simulink model "cblocks"  (Simulink 6.5)
settings: Solver=ode45  SolverMode=SingleTasking  StartTime=0.0  StopTime=999999  MaxStep=10  RelTol=1e-3  AbsTol=1e-3
undefined symbols (not defined in the file or in its folder): TSAMPLE, Upmax, Upmin
settings Model: Creator=Kostas Tsakalis  LastModifiedBy=Kostas Tsakalis
settings DataIOCC: LimitDataPoints=off  SaveOutput=off  SaveTime=off  SignalLoggingName=sigsOut
settings OptimizationCC: BooleanDataType=off
settings DebuggingCC: SolverPrmCheckMsg=none  MultiTaskDSMMsg=warning  MultiTaskCondExecSysMsg=none  StrictBusMsg=None
settings HardwareCC: TargetUnknown=on
settings RTWCC: IncludeERTFirstTime=on

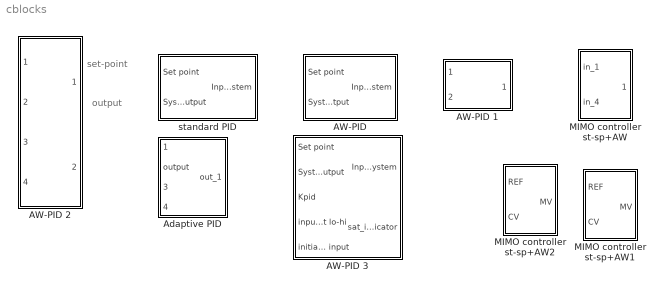
== system cblocks ==
  note: set-point
  note: output
  "AW-PID " : Subsystem  mask(Anti-windup PID ){@1=[.05, 3, 0.5], @2=1/60, @3=0.1, @4=1/60, @5=[0.7 -0.3]}
      mask prompts: @1 "Gain kp - Integral time ki - Derivative time kd"; @2 "Pseudo-derivative filter time constant"; @3 "Error lowpass filter Time constant"; @4 "Sampling Time"; @5 "Saturation Limits [umax umin]"
      mask help: Discrete PID with Anti-windup and with lowpass filter
      mask init:
      | kp=@1(1);ki=@1(2);kd=@1(3);SAM=@2;TF=@3;DT=@4;umax=@5(1);umin=@5(2);
      mask Display: disp('AW-PID+filter')
  AW-PID 1 : Subsystem  mask(Anti-windup PID ){SAM=10, DT=10}
      mask prompts: SAM "Gains: [proportional, Integral, Derivative]"; DT "Pseudo-derivative filter time constant"
      mask help: Discrete PID with Anti-windup
      mask init:
      | kp=@1(1);ki=@1(2);kd=@1(3);umax=@4(1);umin=@4(2);
      mask Display:
      | port_label('output',1,'u')
      | port_label('input',1,'r')
      | port_label('input',2,'y')
  AW-PID 2 : Subsystem  mask(Anti-windup PID ){kpid=[11, 30, 1.5], TCD=.01, TF=0, DT=.01, ipole=0, t_pref=[0.05, 0.4]}
      mask prompts: kpid "PID parameters [kp,ki,kd]"; TCD "Pseudo-derivative filter time constant"; TF "Error lowpass filter Time constant"; DT "Sampling Time"; ipole "Approx. Integrator pole"; t_pref "Reference prefilter [num,den] time constants"
      mask help: Discrete PID with Anti-windup, prefilter, and lowpass filter
      mask init:
      | t_z=t_pref(1);t_p=t_pref(2);
      mask Display:
      | disp('AW-PID+filt ')
      | port_label('input',1,'ref')
      | port_label('input',2,'out')
      | port_label('input',3,'hi')
      | port_label('input',4,'lo')
      | 
      | port_label('output',1,'u')
      | port_label('output',2,'sat')
  AW-PID 3 : Subsystem  mask(Anti-windup PID ){TCD=.01, TF=0, DT=.001, ipole=0}
      mask prompts: TCD "Pseudo-derivative filter time constant"; TF "Error lowpass filter Time constant"; DT "Sampling Time"; ipole "Approx. Integrator pole"
      mask help:
      | Discrete PID with modifications and externalized parameters
      | (adaptation ready).
      | -The PID parameters are externally specified as P,I,D gains (additive form).
      | -Contains externally specified saturation ([lo,hi]) and anti-windup.
      | -Contains an self initializing algorithm, where the value of the 5th input
      | is set as the PID offset u(0).
      | [Typical application to avoid transients: the PID is swithed on with
      | the system at steady state and the system input is connected at u(0)].
      | -Contains a lowpass filter to handle excessive high frequency noise.
      | -Contains an option to modify the integrator pole to a different value
      | to handle problems with zeros at the origin, requiring an unstable
      | compensator.
      mask Display:
      | disp('AW PID \n xtern')
      | port_label('input',1,'ref')
      | port_label('input',2,'y')
      | port_label('input',3,'Kpid')
      | port_label('input',4,'lo-hi')
      | port_label('input',5,'u(0)')
      | 
      | port_label('output',1,'u')
      | port_label('output',2,'sat')
  Adaptive PID : Subsystem
  MIMO controller st-sp+AW : Subsystem
  MIMO controller st-sp+AW1 : Subsystem
  MIMO controller st-sp+AW2 : Subsystem
  standard PID : Subsystem  mask(Discrete PID ){@1=[.05, 3, 0.5], @2=1/60, @3=0.1, @4=1/60}
      mask prompts: @1 "Gain kp - Integral time ki - Derivative time kd"; @2 "Pseudo-derivative filter time constant"; @3 "Error lowpass filter Time constant"; @4 "Sampling Time"
      mask help: Discrete PID with lowpass filter
      mask init:
      | kp=@1(1);ki=@1(2);kd=@1(3);SAM=@2;TF=@3;DT=@4;
      mask Display: disp('PID+filter')

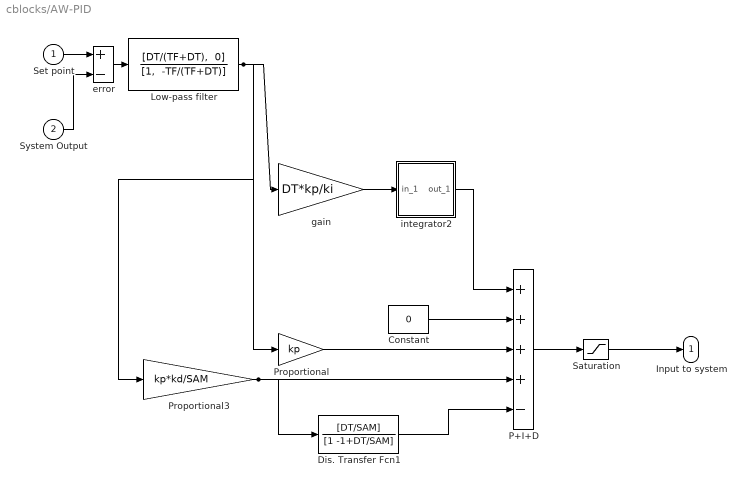
== system cblocks/AW-PID  ==
  Set point : Inport
  System Output : Inport  Port=2
  Constant : Constant  Value=0  OutDataType=sfix(16)  ConRadixGroup=Use specified scaling  OutScaling=2^0  SampleTime=inf  FramePeriod=inf
  Dis. Transfer Fcn1 : DiscreteTransferFcn  Numerator=[DT/SAM]  Denominator=[1 -1+DT/SAM]  SampleTime=DT
  Low-pass filter : DiscreteTransferFcn  Numerator="[DT/(TF+DT),  0]"  Denominator="[1,  -TF/(TF+DT)]"  SampleTime=DT
  P+I+D : Sum  Inputs=++++-  SaturateOnIntegerOverflow=on  InputSameDT=on
  Proportional : Gain  Gain=kp  SaturateOnIntegerOverflow=on
  Proportional3 : Gain  Gain=kp*kd/SAM  SaturateOnIntegerOverflow=on
  Saturation : Saturate  UpperLimit=umax  LowerLimit=umin
  error : Sum  Inputs=+-  SaturateOnIntegerOverflow=on  InputSameDT=on
  gain : Gain  Gain=DT*kp/ki  SaturateOnIntegerOverflow=on
  integrator2 : Subsystem  mask(Anti windup intgrator){@1=umax, @2=umin, @3=DT}
      mask prompts: @1 "umax"; @2 "umin"; @3 "sampling time"
      mask help: Integral with anti-windup
      mask init:
      | umax=@1 ; umin =@2 ;DT=@3;
      mask Display: disp('DT-I-AW')
  Input to system : Outport  InitialOutput=0
  wires:
  Constant/1 -> P+I+D/2
  Saturation/1 -> Input to system/1
  P+I+D/1 -> Saturation/1
  gain/1 -> integrator2/1(in_1)
  Proportional/1 -> P+I+D/3
  Dis. Transfer Fcn1/1 -> P+I+D/5
  Low-pass filter/1 -> gain/1, Proportional3/1, Proportional/1
  Proportional3/1 -> P+I+D/4, Dis. Transfer Fcn1/1
  System Output/1 -> error/2
  Set point/1 -> error/1
  error/1 -> Low-pass filter/1
  integrator2/1(out_1) -> P+I+D/1

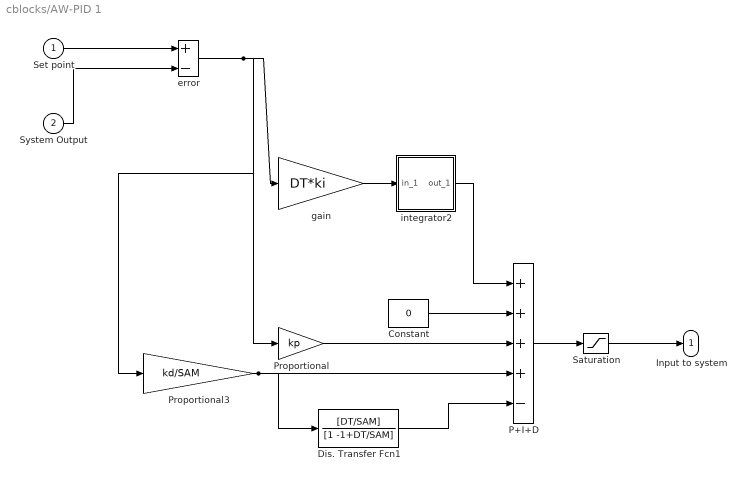
== system cblocks/AW-PID 1 ==
  Set point : Inport
  System Output : Inport  Port=2
  Constant : Constant  Value=0  OutDataType=sfix(16)  ConRadixGroup=Use specified scaling  OutScaling=2^0  SampleTime=inf  FramePeriod=inf
  Dis. Transfer Fcn1 : DiscreteTransferFcn  Numerator=[DT/SAM]  Denominator=[1 -1+DT/SAM]  SampleTime=DT
  P+I+D : Sum  Inputs=++++-  SaturateOnIntegerOverflow=on  InputSameDT=on
  Proportional : Gain  Gain=kp  SaturateOnIntegerOverflow=on
  Proportional3 : Gain  Gain=kd/SAM  SaturateOnIntegerOverflow=on
  Saturation : Saturate  UpperLimit=umax  LowerLimit=umin
  error : Sum  Inputs=+-  SaturateOnIntegerOverflow=on  InputSameDT=on
  gain : Gain  Gain=DT*ki  SaturateOnIntegerOverflow=on
  integrator2 : Subsystem  mask(Anti windup intgrator){@1=umax, @2=umin, @3=DT}
      mask prompts: @1 "umax"; @2 "umin"; @3 "sampling time"
      mask help: Integral with anti-windup
      mask init:
      | umax=@1 ; umin =@2 ;DT=@3;
      mask Display: disp('DT-I-AW')
  Input to system : Outport  InitialOutput=0
  wires:
  Constant/1 -> P+I+D/2
  Saturation/1 -> Input to system/1
  P+I+D/1 -> Saturation/1
  gain/1 -> integrator2/1(in_1)
  Proportional/1 -> P+I+D/3
  Dis. Transfer Fcn1/1 -> P+I+D/5
  Proportional3/1 -> P+I+D/4, Dis. Transfer Fcn1/1
  System Output/1 -> error/2
  Set point/1 -> error/1
  error/1 -> gain/1, Proportional3/1, Proportional/1
  integrator2/1(out_1) -> P+I+D/1

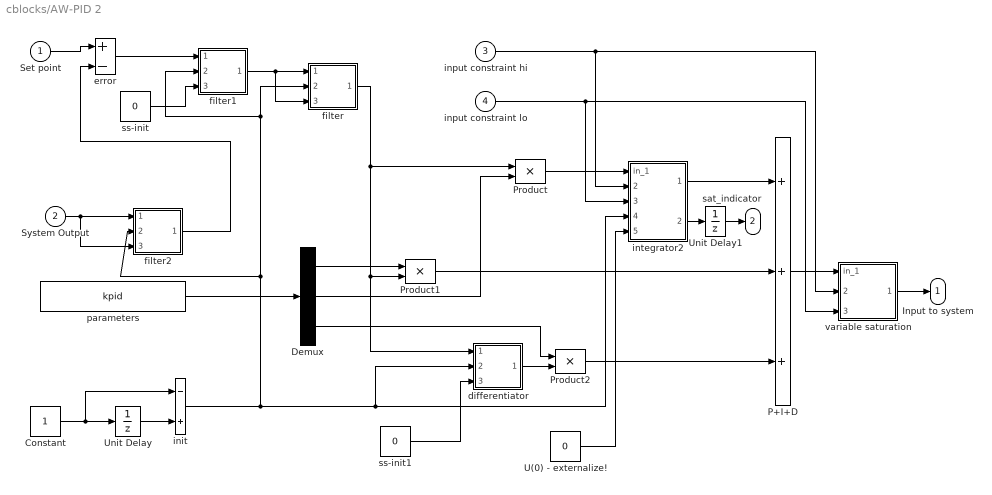
== system cblocks/AW-PID 2 ==
  Set point : Inport
  System Output : Inport  Port=2
  input constraint hi : Inport  Port=3
  input constraint lo : Inport  Port=4
  Constant : Constant  Value=1  OutDataType=sfix(16)  ConRadixGroup=Use specified scaling  OutScaling=2^0  SampleTime=inf  FramePeriod=inf
  Demux : Demux  Outputs=3
  P+I+D : Sum  Inputs=+++  SaturateOnIntegerOverflow=on  InputSameDT=on
  Product : Product  SaturateOnIntegerOverflow=on  InputSameDT=on
  Product1 : Product  SaturateOnIntegerOverflow=on  InputSameDT=on
  Product2 : Product  SaturateOnIntegerOverflow=on  InputSameDT=on
  U(0) - externalize! : Constant  Value=0  OutDataType=sfix(16)  ConRadixGroup=Use specified scaling  OutScaling=2^0  SampleTime=inf  FramePeriod=inf
  Unit Delay : UnitDelay  SampleTime=DT
  Unit Delay1 : UnitDelay  SampleTime=DT
  differentiator : Subsystem  mask(Approx. Differentator){DT=DT, TC=TCD}
      mask prompts: DT "sampling time"; TC "Time constant"
  error : Sum  Inputs=+-  SaturateOnIntegerOverflow=on  InputSameDT=on
  filter : Subsystem  mask(Lead-Lag Filter){DT=DT, TC=TF, TZ=0}
      mask prompts: DT "sampling time"; TC "Pole Time constant"; TZ "Zero Time Constant"
  filter1 : Subsystem  mask(Lead-Lag Filter){DT=DT, TC=t_p, TZ=t_z}
      mask prompts: DT "sampling time"; TC "Pole Time constant"; TZ "Zero Time Constant"
  filter2 : Subsystem  mask(Lead-Lag Filter){DT=DT, TC=t_z, TZ=t_p}
      mask prompts: DT "sampling time"; TC "Pole Time constant"; TZ "Zero Time Constant"
  init : Sum  Inputs=-+  SaturateOnIntegerOverflow=on  InputSameDT=on
  integrator2 : Subsystem  mask(Anti windup intgrator){DT=DT, pole=ipole}
      mask prompts: DT "sampling time"
      mask help: Integral with anti-windup
  parameters : Constant  Value=kpid  OutDataType=sfix(16)  ConRadixGroup=Use specified scaling  OutScaling=2^0  SampleTime=inf  FramePeriod=inf
  ss-init : Constant  Value=0  OutDataType=sfix(16)  ConRadixGroup=Use specified scaling  OutScaling=2^0  SampleTime=inf  FramePeriod=inf
  ss-init1 : Constant  Value=0  OutDataType=sfix(16)  ConRadixGroup=Use specified scaling  OutScaling=2^0  SampleTime=inf  FramePeriod=inf
  variable saturation : Subsystem  mask(Anti windup intgrator){DT=DT}
      mask prompts: DT "sampling time"
      mask help: Integral with anti-windup
      mask Display: disp('DT-I-AW')
  Input to system : Outport  InitialOutput=0
  sat_indicator : Outport  Port=2  InitialOutput=0
  wires:
  Unit Delay1/1 -> sat_indicator/1
  ss-init1/1 -> differentiator/3(init val)
  ss-init/1 -> filter1/3(init val)
  U(0) - externalize!/1 -> integrator2/5(init val)
  integrator2/2(out_2) -> Unit Delay1/1
  init/1 -> filter1/2(init flag), filter/2(init flag), filter2/2(init flag), integrator2/4(init flag), differentiator/2(init flag)
  Unit Delay/1 -> init/2
  Constant/1 -> init/1, Unit Delay/1
  filter/1(out_1) -> differentiator/1(in_1), Product1/2, Product/1
  differentiator/1(out_1) -> Product2/2
  Demux/3 -> Product2/1
  Product1/1 -> P+I+D/2
  Set point/1 -> error/1
  parameters/1 -> Demux/1
  error/1 -> filter1/1(in_1)
  integrator2/1(out_1) -> P+I+D/1
  P+I+D/1 -> variable saturation/1(in_1)
  Product/1 -> integrator2/1(in_1)
  Demux/1 -> Product1/1
  Demux/2 -> Product/2
  Product2/1 -> P+I+D/3
  filter1/1(out_1) -> filter/3(init val), filter/1(in_1)
  System Output/1 -> filter2/3(init val), filter2/1(in_1)
  filter2/1(out_1) -> error/2
  variable saturation/1(out_1) -> Input to system/1
  input constraint lo/1 -> integrator2/3(umin), variable saturation/3(umin)
  input constraint hi/1 -> integrator2/2(umax), variable saturation/2(umax)

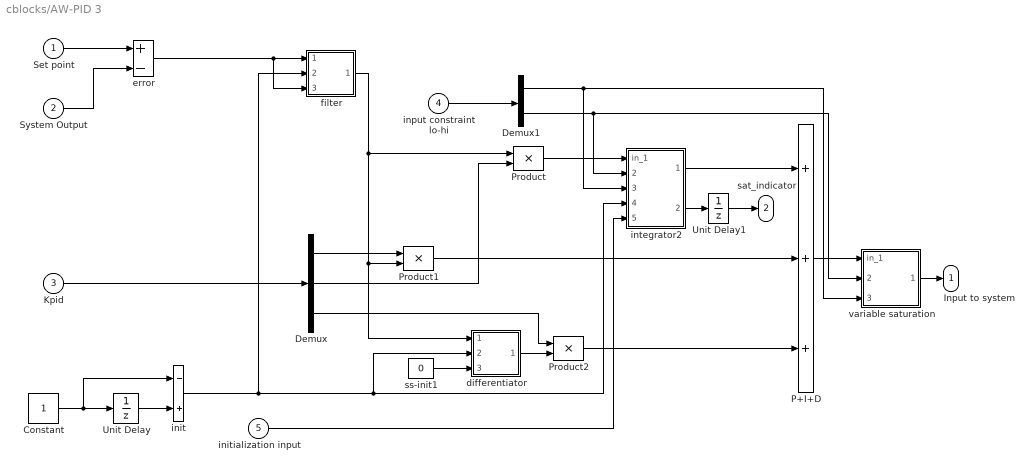
== system cblocks/AW-PID 3 ==
  Set point : Inport
  System Output : Inport  Port=2
  Kpid : Inport  Port=3
  input constraint lo-hi : Inport  Port=4
  initialization input : Inport  Port=5
  Constant : Constant  Value=1  OutDataType=sfix(16)  ConRadixGroup=Use specified scaling  OutScaling=2^0  SampleTime=inf  FramePeriod=inf
  Demux : Demux  Outputs=3
  Demux1 : Demux  Outputs=2
  P+I+D : Sum  Inputs=+++  SaturateOnIntegerOverflow=on  InputSameDT=on
  Product : Product  SaturateOnIntegerOverflow=on  InputSameDT=on
  Product1 : Product  SaturateOnIntegerOverflow=on  InputSameDT=on
  Product2 : Product  SaturateOnIntegerOverflow=on  InputSameDT=on
  Unit Delay : UnitDelay  SampleTime=DT
  Unit Delay1 : UnitDelay  SampleTime=DT
  differentiator : Subsystem  mask(Approx. Differentator){DT=DT, TC=TCD}
      mask prompts: DT "sampling time"; TC "Time constant"
  error : Sum  Inputs=+-  SaturateOnIntegerOverflow=on  InputSameDT=on
  filter : Subsystem  mask(Lead-Lag Filter){DT=DT, TC=TF, TZ=0}
      mask prompts: DT "sampling time"; TC "Pole Time constant"; TZ "Zero Time Constant"
  init : Sum  Inputs=-+  SaturateOnIntegerOverflow=on  InputSameDT=on
  integrator2 : Subsystem  mask(Anti windup intgrator){DT=DT, pole=ipole}
      mask prompts: DT "sampling time"
      mask help: Integral with anti-windup
  ss-init1 : Constant  Value=0  OutDataType=sfix(16)  ConRadixGroup=Use specified scaling  OutScaling=2^0  SampleTime=inf  FramePeriod=inf
  variable saturation : Subsystem  mask(Anti windup intgrator){DT=DT}
      mask prompts: DT "sampling time"
      mask help: Integral with anti-windup
      mask Display: disp('DT-I-AW')
  Input to system : Outport  InitialOutput=0
  sat_indicator : Outport  Port=2  InitialOutput=0
  wires:
  Demux1/2 -> integrator2/2(umax), variable saturation/2(umax)
  input constraint lo-hi/1 -> Demux1/1
  System Output/1 -> error/2
  Unit Delay1/1 -> sat_indicator/1
  ss-init1/1 -> differentiator/3(init val)
  initialization input/1 -> integrator2/5(init val)
  integrator2/2(out_2) -> Unit Delay1/1
  init/1 -> filter/2(init flag), integrator2/4(init flag), differentiator/2(init flag)
  Unit Delay/1 -> init/2
  Constant/1 -> init/1, Unit Delay/1
  filter/1(out_1) -> differentiator/1(in_1), Product1/2, Product/1
  differentiator/1(out_1) -> Product2/2
  Demux/3 -> Product2/1
  Product1/1 -> P+I+D/2
  Set point/1 -> error/1
  Kpid/1 -> Demux/1
  error/1 -> filter/3(init val), filter/1(in_1)
  integrator2/1(out_1) -> P+I+D/1
  P+I+D/1 -> variable saturation/1(in_1)
  Product/1 -> integrator2/1(in_1)
  Demux/1 -> Product1/1
  Demux/2 -> Product/2
  Product2/1 -> P+I+D/3
  variable saturation/1(out_1) -> Input to system/1
  Demux1/1 -> integrator2/3(umin), variable saturation/3(umin)

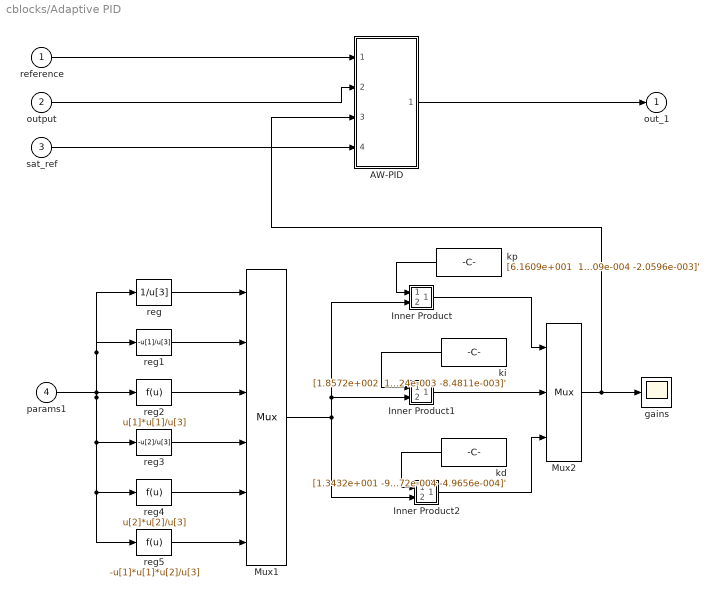
== system cblocks/Adaptive PID ==
  reference : Inport
  output : Inport  Port=2
  sat_ref : Inport  Port=3
  params1 : Inport  Port=4
  "AW-PID " : Subsystem  mask(Anti-windup PID ){SAM=.02, TF=.02, DT=.02}
      mask prompts: SAM "Pseudo-derivative filter time constant"; TF "Error lowpass filter Time constant"; DT "Sampling Time"
      mask help: Discrete PID with Anti-windup and with lowpass filter
      mask init:
      | umax=@4(1);umin=@4(2);t_z=@5(1);t_p=@5(2);
      mask Display: disp('Adaptive\n AW-PID\n+filter')
  Inner Product : Subsystem
      mask Type: Dot Product
      mask Description:
      | Inner (dot) product.
      | y=sum(u1.*u2)
      mask Help: Computes the inner (dot) product of the inputs: sum(u1.*u2).  The inputs are vectors of the same length. Output is a scalar.
      mask Display: disp('.\n')
  Inner Product1 : Subsystem
      mask Type: Dot Product
      mask Description:
      | Inner (dot) product.
      | y=sum(u1.*u2)
      mask Help: Computes the inner (dot) product of the inputs: sum(u1.*u2).  The inputs are vectors of the same length. Output is a scalar.
      mask Display: disp('.\n')
  Inner Product2 : Subsystem
      mask Type: Dot Product
      mask Description:
      | Inner (dot) product.
      | y=sum(u1.*u2)
      mask Help: Computes the inner (dot) product of the inputs: sum(u1.*u2).  The inputs are vectors of the same length. Output is a scalar.
      mask Display: disp('.\n')
  Mux1 : Mux  Inputs=6
  Mux2 : Mux  Inputs=3
  gains : Scope
      settings: TickLabels=on  YMin=0  YMax=325  DataFormat=Array  MaxDataPoints=10000
  kd : Constant  Orientation=left  Value="[1.3432e+001 -9.0958e-001  6.3780e-002  2.0466e-001 -2.8572e-004 -4.9656e-004]'"  OutDataType=sfix(16)  ConRadixGroup=Use specified scaling  OutScaling=2^0  SampleTime=inf  FramePeriod=inf
  ki : Constant  Orientation=left  Value="[1.8572e+002  1.4910e+000  1.1727e+000  3.6398e+000  1.2924e-003 -8.4811e-003]'"  OutDataType=sfix(16)  ConRadixGroup=Use specified scaling  OutScaling=2^0  SampleTime=inf  FramePeriod=inf
  kp : Constant  Orientation=left  Value="[6.1609e+001  1.3054e+000  2.8868e-001  2.0449e+000 -3.9509e-004 -2.0596e-003]'"  OutDataType=sfix(16)  ConRadixGroup=Use specified scaling  OutScaling=2^0  SampleTime=inf  FramePeriod=inf
  reg : Fcn  Expr=1/u[3]
  reg1 : Fcn  Expr=-u[1]/u[3]
  reg2 : Fcn  Expr=u[1]*u[1]/u[3]
  reg3 : Fcn  Expr=-u[2]/u[3]
  reg4 : Fcn  Expr=u[2]*u[2]/u[3]
  reg5 : Fcn  Expr=-u[1]*u[1]*u[2]/u[3]
  out_1 : Outport  InitialOutput=0
  wires:
  sat_ref/1 -> "AW-PID "/4(input constraint)
  reference/1 -> "AW-PID "/1(Set point)
  "AW-PID "/1(Input to system) -> out_1/1
  params1/1 -> reg/1, reg1/1, reg2/1, reg3/1, reg4/1, reg5/1
  reg5/1 -> Mux1/6
  reg4/1 -> Mux1/5
  reg3/1 -> Mux1/4
  reg2/1 -> Mux1/3
  reg1/1 -> Mux1/2
  reg/1 -> Mux1/1
  Mux1/1 -> Inner Product2/2(in_2), Inner Product1/2(in_2), Inner Product/2(in_2)
  Inner Product1/1(out_1) -> Mux2/2
  Inner Product/1(out_1) -> Mux2/1
  Inner Product2/1(out_1) -> Mux2/3
  kp/1 -> Inner Product/1(in_1)
  ki/1 -> Inner Product1/1(in_1)
  kd/1 -> Inner Product2/1(in_1)
  Mux2/1 -> gains/1, "AW-PID "/3(parameters)
  output/1 -> "AW-PID "/2(System Output)

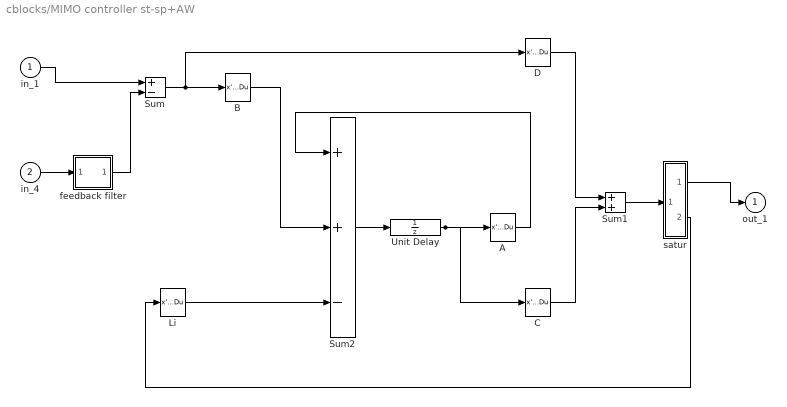
== system cblocks/MIMO controller st-sp+AW ==
  in_1 : Inport
  in_4 : Inport  Port=2
  A : StateSpace  A=[]  B=[]  C=[]  D=K  mask(Matrix Gain){@1=Aci}
      mask prompts: @1 "Gain matrix:"
      mask help: Matrix Gain.
      mask init:
      | K = @1;
      mask Help: Multiplies input vector by entered matrix to produce output vector (y=Au).
      mask Display: disp('K')
  B : StateSpace  A=[]  B=[]  C=[]  D=K  mask(Matrix Gain){@1=Bci}
      mask prompts: @1 "Gain matrix:"
      mask help: Matrix Gain.
      mask init:
      | K = @1;
      mask Help: Multiplies input vector by entered matrix to produce output vector (y=Au).
      mask Display: disp('K')
  C : StateSpace  A=[]  B=[]  C=[]  D=K  mask(Matrix Gain){@1=Cci}
      mask prompts: @1 "Gain matrix:"
      mask help: Matrix Gain.
      mask init:
      | K = @1;
      mask Help: Multiplies input vector by entered matrix to produce output vector (y=Au).
      mask Display: disp('K')
  D : StateSpace  A=[]  B=[]  C=[]  D=K  mask(Matrix Gain){@1=Dci}
      mask prompts: @1 "Gain matrix:"
      mask help: Matrix Gain.
      mask init:
      | K = @1;
      mask Help: Multiplies input vector by entered matrix to produce output vector (y=Au).
      mask Display: disp('K')
  Li : StateSpace  A=[]  B=[]  C=[]  D=K  mask(Matrix Gain){@1=LDi}
      mask prompts: @1 "Gain matrix:"
      mask help: Matrix Gain.
      mask init:
      | K = @1;
      mask Help: Multiplies input vector by entered matrix to produce output vector (y=Au).
      mask Display: disp('K')
  Sum : Sum  Inputs=+-  SaturateOnIntegerOverflow=on  InputSameDT=on
  Sum1 : Sum  SaturateOnIntegerOverflow=on  InputSameDT=on
  Sum2 : Sum  Inputs=++-  SaturateOnIntegerOverflow=on  InputSameDT=on
  Unit Delay : UnitDelay  SampleTime=TSAMPLE
  feedback filter : Subsystem
  satur : Subsystem  mask(saturations and dead zones){@1=[1 1 1], @2=[0 0 0]}
      mask prompts: @1 "max 1-2-3"; @2 "min 1-2-3"
      mask help: sats+dzn
      mask init:
      | Upmax=@1;Upmin=@2;
  out_1 : Outport  InitialOutput=0
  wires:
  in_1/1 -> Sum/1
  Sum/1 -> B/1, D/1
  D/1 -> Sum1/1
  Sum2/1 -> Unit Delay/1
  A/1 -> Sum2/1
  B/1 -> Sum2/2
  C/1 -> Sum1/2
  Unit Delay/1 -> A/1, C/1
  Li/1 -> Sum2/3
  Sum1/1 -> satur/1(in_1)
  satur/1(out_1) -> out_1/1
  satur/2(out_2) -> Li/1
  in_4/1 -> feedback filter/1(in_1)
  feedback filter/1(out_1) -> Sum/2

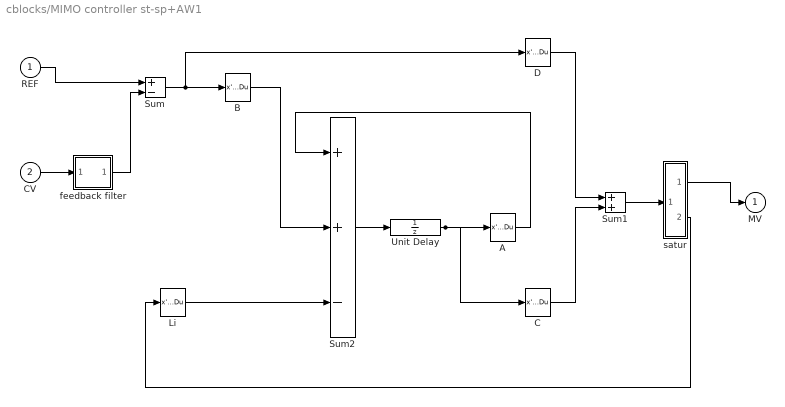
== system cblocks/MIMO controller st-sp+AW1 ==
  REF : Inport
  CV : Inport  Port=2
  A : StateSpace  A=[]  B=[]  C=[]  D=K  mask(Matrix Gain){@1=Aci}
      mask prompts: @1 "Gain matrix:"
      mask help: Matrix Gain.
      mask init:
      | K = @1;
      mask Help: Multiplies input vector by entered matrix to produce output vector (y=Au).
      mask Display: disp('K')
  B : StateSpace  A=[]  B=[]  C=[]  D=K  mask(Matrix Gain){@1=Bci}
      mask prompts: @1 "Gain matrix:"
      mask help: Matrix Gain.
      mask init:
      | K = @1;
      mask Help: Multiplies input vector by entered matrix to produce output vector (y=Au).
      mask Display: disp('K')
  C : StateSpace  A=[]  B=[]  C=[]  D=K  mask(Matrix Gain){@1=Cci}
      mask prompts: @1 "Gain matrix:"
      mask help: Matrix Gain.
      mask init:
      | K = @1;
      mask Help: Multiplies input vector by entered matrix to produce output vector (y=Au).
      mask Display: disp('K')
  D : StateSpace  A=[]  B=[]  C=[]  D=K  mask(Matrix Gain){@1=Dci}
      mask prompts: @1 "Gain matrix:"
      mask help: Matrix Gain.
      mask init:
      | K = @1;
      mask Help: Multiplies input vector by entered matrix to produce output vector (y=Au).
      mask Display: disp('K')
  Li : StateSpace  A=[]  B=[]  C=[]  D=K  mask(Matrix Gain){@1=LDi}
      mask prompts: @1 "Gain matrix:"
      mask help: Matrix Gain.
      mask init:
      | K = @1;
      mask Help: Multiplies input vector by entered matrix to produce output vector (y=Au).
      mask Display: disp('K')
  Sum : Sum  Inputs=+-  SaturateOnIntegerOverflow=on  InputSameDT=on
  Sum1 : Sum  SaturateOnIntegerOverflow=on  InputSameDT=on
  Sum2 : Sum  Inputs=++-  SaturateOnIntegerOverflow=on  InputSameDT=on
  Unit Delay : UnitDelay  SampleTime=TSAMPLE
  feedback filter : Subsystem
  satur : Subsystem  mask(saturations and dead zones){@1=Upmax, @2=Upmin}
      mask prompts: @1 "max 1-2-3"; @2 "min 1-2-3"
      mask help: sats+dzn
      mask init:
      | Upmax=@1;Upmin=@2;
  MV : Outport  InitialOutput=0
  wires:
  REF/1 -> Sum/1
  Sum/1 -> B/1, D/1
  D/1 -> Sum1/1
  Sum2/1 -> Unit Delay/1
  A/1 -> Sum2/1
  B/1 -> Sum2/2
  C/1 -> Sum1/2
  Unit Delay/1 -> A/1, C/1
  Li/1 -> Sum2/3
  Sum1/1 -> satur/1(in_1)
  satur/1(out_1) -> MV/1
  satur/2(out_2) -> Li/1
  CV/1 -> feedback filter/1(in_1)
  feedback filter/1(out_1) -> Sum/2

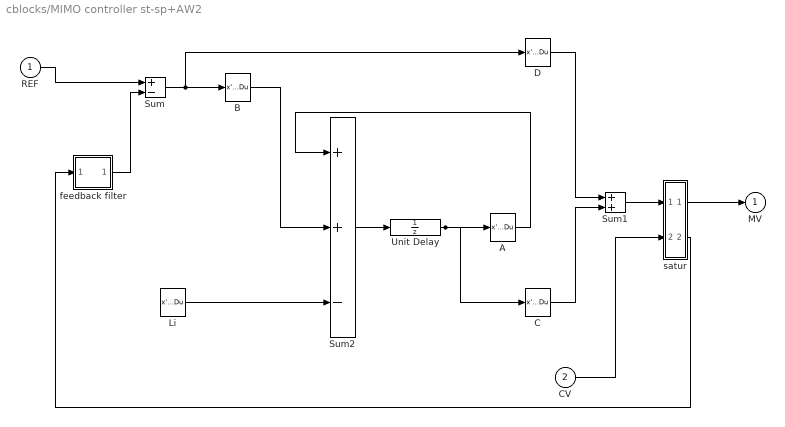
== system cblocks/MIMO controller st-sp+AW2 ==
  REF : Inport
  CV : Inport  Port=2
  A : StateSpace  A=[]  B=[]  C=[]  D=K  mask(Matrix Gain){@1=Aci}
      mask prompts: @1 "Gain matrix:"
      mask help: Matrix Gain.
      mask init:
      | K = @1;
      mask Help: Multiplies input vector by entered matrix to produce output vector (y=Au).
      mask Display: disp('K')
  B : StateSpace  A=[]  B=[]  C=[]  D=K  mask(Matrix Gain){@1=Bci}
      mask prompts: @1 "Gain matrix:"
      mask help: Matrix Gain.
      mask init:
      | K = @1;
      mask Help: Multiplies input vector by entered matrix to produce output vector (y=Au).
      mask Display: disp('K')
  C : StateSpace  A=[]  B=[]  C=[]  D=K  mask(Matrix Gain){@1=Cci}
      mask prompts: @1 "Gain matrix:"
      mask help: Matrix Gain.
      mask init:
      | K = @1;
      mask Help: Multiplies input vector by entered matrix to produce output vector (y=Au).
      mask Display: disp('K')
  D : StateSpace  A=[]  B=[]  C=[]  D=K  mask(Matrix Gain){@1=Dci}
      mask prompts: @1 "Gain matrix:"
      mask help: Matrix Gain.
      mask init:
      | K = @1;
      mask Help: Multiplies input vector by entered matrix to produce output vector (y=Au).
      mask Display: disp('K')
  Li : StateSpace  A=[]  B=[]  C=[]  D=K  mask(Matrix Gain){@1=LDi}
      mask prompts: @1 "Gain matrix:"
      mask help: Matrix Gain.
      mask init:
      | K = @1;
      mask Help: Multiplies input vector by entered matrix to produce output vector (y=Au).
      mask Display: disp('K')
  Sum : Sum  Inputs=+-  SaturateOnIntegerOverflow=on  InputSameDT=on
  Sum1 : Sum  SaturateOnIntegerOverflow=on  InputSameDT=on
  Sum2 : Sum  Inputs=++-  SaturateOnIntegerOverflow=on  InputSameDT=on
  Unit Delay : UnitDelay  SampleTime=TSAMPLE
  feedback filter : Subsystem
  satur : Subsystem
  MV : Outport  InitialOutput=0
  wires:
  satur/2(ysadjust) -> feedback filter/1(in_1)
  CV/1 -> satur/2(ys)
  REF/1 -> Sum/1
  Sum/1 -> B/1, D/1
  D/1 -> Sum1/1
  Sum2/1 -> Unit Delay/1
  A/1 -> Sum2/1
  B/1 -> Sum2/2
  C/1 -> Sum1/2
  Unit Delay/1 -> A/1, C/1
  Li/1 -> Sum2/3
  Sum1/1 -> satur/1(u_desired)
  satur/1(power) -> MV/1
  feedback filter/1(out_1) -> Sum/2

== system cblocks/standard PID ==
  Set point : Inport
  System Output : Inport  Port=2
  Constant : Constant  Value=0  OutDataType=sfix(16)  ConRadixGroup=Use specified scaling  OutScaling=2^0  SampleTime=inf  FramePeriod=inf
  Dis. Transfer Fcn1 : DiscreteTransferFcn  Numerator=[DT/SAM]  Denominator=[1 -1+DT/SAM]  SampleTime=DT
  Low-pass filter : DiscreteTransferFcn  Numerator="[DT/(TF+DT),  0]"  Denominator=[1 -TF/(TF+DT)]  SampleTime=DT
  P+I+D : Sum  Inputs=++++-  SaturateOnIntegerOverflow=on  InputSameDT=on
  Proportional : Gain  Gain=kp  SaturateOnIntegerOverflow=on
  Proportional3 : Gain  Gain=kp*kd/SAM  SaturateOnIntegerOverflow=on
  error : Sum  Inputs=+-  SaturateOnIntegerOverflow=on  InputSameDT=on
  gain : Gain  Gain=DT*kp/ki  SaturateOnIntegerOverflow=on
  integrator1 : Subsystem
  Input to system : Outport  InitialOutput=0
  wires:
  Constant/1 -> P+I+D/2
  gain/1 -> integrator1/1(in_1)
  Proportional/1 -> P+I+D/3
  Dis. Transfer Fcn1/1 -> P+I+D/5
  Low-pass filter/1 -> gain/1, Proportional3/1, Proportional/1
  Proportional3/1 -> P+I+D/4, Dis. Transfer Fcn1/1
  System Output/1 -> error/2
  Set point/1 -> error/1
  error/1 -> Low-pass filter/1
  integrator1/1(out_1) -> P+I+D/1
  P+I+D/1 -> Input to system/1

== system cblocks/AW-PID /integrator2 ==
  in_1 : Inport
  Constant : Constant  Value=umax  OutDataType=sfix(16)  ConRadixGroup=Use specified scaling  OutScaling=2^0  SampleTime=inf  FramePeriod=inf
  Constant3 : Constant  Value=umin  OutDataType=sfix(16)  ConRadixGroup=Use specified scaling  OutScaling=2^0  SampleTime=inf  FramePeriod=inf
  Switch : Switch  SaturateOnIntegerOverflow=on  InputSameDT=on
  Switch2 : Switch  SaturateOnIntegerOverflow=on  InputSameDT=on
  delay : DiscreteTransferFcn  Orientation=left  Denominator=[1 0]  SampleTime=DT
  error1 : Sum  SaturateOnIntegerOverflow=on  InputSameDT=on
  error2 : Sum  Inputs=+-  SaturateOnIntegerOverflow=on  InputSameDT=on
  error3 : Sum  Inputs=+-  SaturateOnIntegerOverflow=on  InputSameDT=on
  out_1 : Outport  InitialOutput=0
  wires:
  in_1/1 -> error1/2
  Switch2/1 -> out_1/1, delay/1
  Switch/1 -> Switch2/1, error3/1
  Constant3/1 -> Switch2/3, error3/2
  error3/1 -> Switch2/2
  error1/1 -> Switch/1, error2/2
  Constant/1 -> Switch/3, error2/1
  error2/1 -> Switch/2
  delay/1 -> error1/1

== system cblocks/AW-PID 1/integrator2 ==
  in_1 : Inport
  Constant : Constant  Value=umax  OutDataType=sfix(16)  ConRadixGroup=Use specified scaling  OutScaling=2^0  SampleTime=inf  FramePeriod=inf
  Constant3 : Constant  Value=umin  OutDataType=sfix(16)  ConRadixGroup=Use specified scaling  OutScaling=2^0  SampleTime=inf  FramePeriod=inf
  Switch : Switch  SaturateOnIntegerOverflow=on  InputSameDT=on
  Switch2 : Switch  SaturateOnIntegerOverflow=on  InputSameDT=on
  delay : DiscreteTransferFcn  Orientation=left  Denominator=[1 0]  SampleTime=DT
  error1 : Sum  SaturateOnIntegerOverflow=on  InputSameDT=on
  error2 : Sum  Inputs=+-  SaturateOnIntegerOverflow=on  InputSameDT=on
  error3 : Sum  Inputs=+-  SaturateOnIntegerOverflow=on  InputSameDT=on
  out_1 : Outport  InitialOutput=0
  wires:
  in_1/1 -> error1/2
  Switch2/1 -> out_1/1, delay/1
  Switch/1 -> Switch2/1, error3/1
  Constant3/1 -> Switch2/3, error3/2
  error3/1 -> Switch2/2
  error1/1 -> Switch/1, error2/2
  Constant/1 -> Switch/3, error2/1
  error2/1 -> Switch/2
  delay/1 -> error1/1

== system cblocks/AW-PID 2/differentiator ==
  in_1 : Inport
  init flag : Inport  Port=2
  init val : Inport  Port=3
  Switch1 : Switch  SaturateOnIntegerOverflow=on  InputSameDT=on
  Switch2 : Switch  SaturateOnIntegerOverflow=on  InputSameDT=on
  Unit Delay : UnitDelay  Orientation=left  SampleTime=DT
  Unit Delay1 : UnitDelay  SampleTime=DT
  error1 : Sum  Inputs=++-  SaturateOnIntegerOverflow=on  InputSameDT=on
  gain : Gain  Gain=1/(DT+TC)  SaturateOnIntegerOverflow=on
  gain1 : Gain  Orientation=left  Gain=TC/(TC+DT)  SaturateOnIntegerOverflow=on
  out_1 : Outport  InitialOutput=0
  wires:
  gain1/1 -> error1/1
  Switch2/1 -> error1/3
  Unit Delay1/1 -> Switch2/1
  Unit Delay/1 -> gain1/1
  gain/1 -> error1/2, Switch2/3, Unit Delay1/1
  in_1/1 -> gain/1
  Switch1/1 -> Unit Delay/1, out_1/1
  error1/1 -> Switch1/1
  init flag/1 -> Switch2/2, Switch1/2
  init val/1 -> Switch1/3

== system cblocks/AW-PID 2/filter ==
  in_1 : Inport
  init flag : Inport  Port=2
  init val : Inport  Port=3
  Switch1 : Switch  SaturateOnIntegerOverflow=on  InputSameDT=on
  Switch2 : Switch  SaturateOnIntegerOverflow=on  InputSameDT=on
  Unit Delay : UnitDelay  Orientation=left  SampleTime=DT
  Unit Delay1 : UnitDelay  SampleTime=DT
  error1 : Sum  Inputs=+++-  SaturateOnIntegerOverflow=on  InputSameDT=on
  gain : Gain  Gain=TZ/(DT+TC)  SaturateOnIntegerOverflow=on
  gain1 : Gain  Orientation=left  Gain=TC/(TC+DT)  SaturateOnIntegerOverflow=on
  gain2 : Gain  Gain=DT/(DT+TC)  SaturateOnIntegerOverflow=on
  out_1 : Outport  InitialOutput=0
  wires:
  gain2/1 -> error1/2
  init val/1 -> Switch1/3
  init flag/1 -> Switch1/2, Switch2/2
  error1/1 -> Switch1/1
  Switch1/1 -> out_1/1, Unit Delay/1
  in_1/1 -> gain2/1, gain/1
  gain/1 -> Unit Delay1/1, Switch2/3, error1/3
  Unit Delay/1 -> gain1/1
  Unit Delay1/1 -> Switch2/1
  Switch2/1 -> error1/4
  gain1/1 -> error1/1

== system cblocks/AW-PID 2/filter1 ==
  in_1 : Inport
  init flag : Inport  Port=2
  init val : Inport  Port=3
  Switch1 : Switch  SaturateOnIntegerOverflow=on  InputSameDT=on
  Switch2 : Switch  SaturateOnIntegerOverflow=on  InputSameDT=on
  Unit Delay : UnitDelay  Orientation=left  SampleTime=DT
  Unit Delay1 : UnitDelay  SampleTime=DT
  error1 : Sum  Inputs=+++-  SaturateOnIntegerOverflow=on  InputSameDT=on
  gain : Gain  Gain=TZ/(DT+TC)  SaturateOnIntegerOverflow=on
  gain1 : Gain  Orientation=left  Gain=TC/(TC+DT)  SaturateOnIntegerOverflow=on
  gain2 : Gain  Gain=DT/(DT+TC)  SaturateOnIntegerOverflow=on
  out_1 : Outport  InitialOutput=0
  wires:
  gain1/1 -> error1/1
  Switch2/1 -> error1/4
  Unit Delay1/1 -> Switch2/1
  Unit Delay/1 -> gain1/1
  gain/1 -> error1/3, Switch2/3, Unit Delay1/1
  in_1/1 -> gain/1, gain2/1
  Switch1/1 -> Unit Delay/1, out_1/1
  error1/1 -> Switch1/1
  init flag/1 -> Switch2/2, Switch1/2
  init val/1 -> Switch1/3
  gain2/1 -> error1/2

== system cblocks/AW-PID 2/filter2 ==
  in_1 : Inport
  init flag : Inport  Port=2
  init val : Inport  Port=3
  Switch1 : Switch  SaturateOnIntegerOverflow=on  InputSameDT=on
  Switch2 : Switch  SaturateOnIntegerOverflow=on  InputSameDT=on
  Unit Delay : UnitDelay  Orientation=left  SampleTime=DT
  Unit Delay1 : UnitDelay  SampleTime=DT
  error1 : Sum  Inputs=+++-  SaturateOnIntegerOverflow=on  InputSameDT=on
  gain : Gain  Gain=TZ/(DT+TC)  SaturateOnIntegerOverflow=on
  gain1 : Gain  Orientation=left  Gain=TC/(TC+DT)  SaturateOnIntegerOverflow=on
  gain2 : Gain  Gain=DT/(DT+TC)  SaturateOnIntegerOverflow=on
  out_1 : Outport  InitialOutput=0
  wires:
  gain2/1 -> error1/2
  init val/1 -> Switch1/3
  init flag/1 -> Switch1/2, Switch2/2
  error1/1 -> Switch1/1
  Switch1/1 -> out_1/1, Unit Delay/1
  in_1/1 -> gain2/1, gain/1
  gain/1 -> Unit Delay1/1, Switch2/3, error1/3
  Unit Delay/1 -> gain1/1
  Unit Delay1/1 -> Switch2/1
  Switch2/1 -> error1/4
  gain1/1 -> error1/1

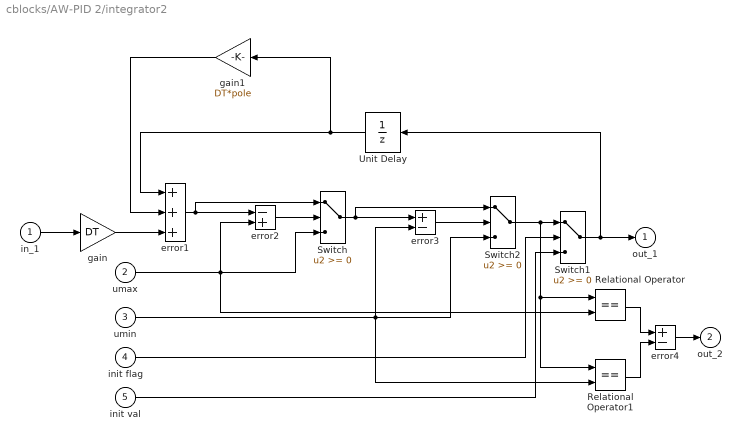
== system cblocks/AW-PID 2/integrator2 ==
  in_1 : Inport
  umax : Inport  Port=2
  umin : Inport  Port=3
  init flag : Inport  Port=4
  init val : Inport  Port=5
  Relational Operator : RelationalOperator  Operator===  InputSameDT=on
  Relational Operator1 : RelationalOperator  Operator===  InputSameDT=on
  Switch : Switch  SaturateOnIntegerOverflow=on  InputSameDT=on
  Switch1 : Switch  SaturateOnIntegerOverflow=on  InputSameDT=on
  Switch2 : Switch  SaturateOnIntegerOverflow=on  InputSameDT=on
  Unit Delay : UnitDelay  Orientation=left  SampleTime=DT
  error1 : Sum  Inputs=+++  SaturateOnIntegerOverflow=on  InputSameDT=on
  error2 : Sum  Inputs=-+  SaturateOnIntegerOverflow=on  InputSameDT=on
  error3 : Sum  Inputs=+-  SaturateOnIntegerOverflow=on  InputSameDT=on
  error4 : Sum  Inputs=+-  SaturateOnIntegerOverflow=on  InputSameDT=on
  gain : Gain  Gain=DT  SaturateOnIntegerOverflow=on
  gain1 : Gain  Orientation=left  Gain=DT*pole  SaturateOnIntegerOverflow=on
  out_1 : Outport  InitialOutput=0
  out_2 : Outport  Port=2  InitialOutput=0
  wires:
  Unit Delay/1 -> gain1/1, error1/1
  error4/1 -> out_2/1
  Relational Operator/1 -> error4/1
  Relational Operator1/1 -> error4/2
  Switch/1 -> Switch2/1, error3/1
  init val/1 -> Switch1/3
  init flag/1 -> Switch1/2
  Switch2/1 -> Relational Operator1/1, Relational Operator/1, Switch1/1
  Switch1/1 -> Unit Delay/1, out_1/1
  gain1/1 -> error1/2
  gain/1 -> error1/3
  error2/1 -> Switch/2
  error3/1 -> Switch2/2
  umin/1 -> Relational Operator1/2, error3/2, Switch2/3
  umax/1 -> Relational Operator/2, error2/2, Switch/3
  error1/1 -> error2/1, Switch/1
  in_1/1 -> gain/1

== system cblocks/AW-PID 2/variable saturation ==
  in_1 : Inport
  umax : Inport  Port=2
  umin : Inport  Port=3
  Switch : Switch  SaturateOnIntegerOverflow=on  InputSameDT=on
  Switch2 : Switch  SaturateOnIntegerOverflow=on  InputSameDT=on
  error2 : Sum  Inputs=+-  SaturateOnIntegerOverflow=on  InputSameDT=on
  error3 : Sum  Inputs=+-  SaturateOnIntegerOverflow=on  InputSameDT=on
  out_1 : Outport  InitialOutput=0
  wires:
  in_1/1 -> Switch/1, error2/2
  Switch2/1 -> out_1/1
  Switch/1 -> Switch2/1, error3/1
  umax/1 -> Switch/3, error2/1
  umin/1 -> Switch2/3, error3/2
  error3/1 -> Switch2/2
  error2/1 -> Switch/2

== system cblocks/AW-PID 3/differentiator ==
  in_1 : Inport
  init flag : Inport  Port=2
  init val : Inport  Port=3
  Switch1 : Switch  SaturateOnIntegerOverflow=on  InputSameDT=on
  Switch2 : Switch  SaturateOnIntegerOverflow=on  InputSameDT=on
  Unit Delay : UnitDelay  Orientation=left  SampleTime=DT
  Unit Delay1 : UnitDelay  SampleTime=DT
  error1 : Sum  Inputs=++-  SaturateOnIntegerOverflow=on  InputSameDT=on
  gain : Gain  Gain=1/(DT+TC)  SaturateOnIntegerOverflow=on
  gain1 : Gain  Orientation=left  Gain=TC/(TC+DT)  SaturateOnIntegerOverflow=on
  out_1 : Outport  InitialOutput=0
  wires:
  gain1/1 -> error1/1
  Switch2/1 -> error1/3
  Unit Delay1/1 -> Switch2/1
  Unit Delay/1 -> gain1/1
  gain/1 -> error1/2, Switch2/3, Unit Delay1/1
  in_1/1 -> gain/1
  Switch1/1 -> Unit Delay/1, out_1/1
  error1/1 -> Switch1/1
  init flag/1 -> Switch2/2, Switch1/2
  init val/1 -> Switch1/3

== system cblocks/AW-PID 3/filter ==
  in_1 : Inport
  init flag : Inport  Port=2
  init val : Inport  Port=3
  Switch1 : Switch  SaturateOnIntegerOverflow=on  InputSameDT=on
  Switch2 : Switch  SaturateOnIntegerOverflow=on  InputSameDT=on
  Unit Delay : UnitDelay  Orientation=left  SampleTime=DT
  Unit Delay1 : UnitDelay  SampleTime=DT
  error1 : Sum  Inputs=+++-  SaturateOnIntegerOverflow=on  InputSameDT=on
  gain : Gain  Gain=TZ/(DT+TC)  SaturateOnIntegerOverflow=on
  gain1 : Gain  Orientation=left  Gain=TC/(TC+DT)  SaturateOnIntegerOverflow=on
  gain2 : Gain  Gain=DT/(DT+TC)  SaturateOnIntegerOverflow=on
  out_1 : Outport  InitialOutput=0
  wires:
  gain2/1 -> error1/2
  init val/1 -> Switch1/3
  init flag/1 -> Switch1/2, Switch2/2
  error1/1 -> Switch1/1
  Switch1/1 -> out_1/1, Unit Delay/1
  in_1/1 -> gain2/1, gain/1
  gain/1 -> Unit Delay1/1, Switch2/3, error1/3
  Unit Delay/1 -> gain1/1
  Unit Delay1/1 -> Switch2/1
  Switch2/1 -> error1/4
  gain1/1 -> error1/1

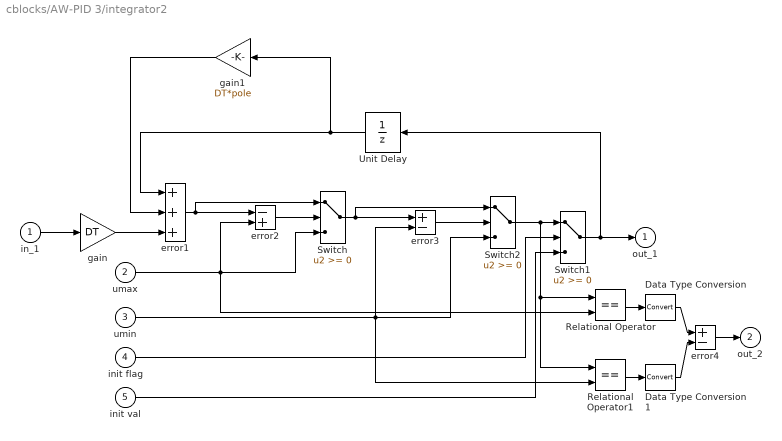
== system cblocks/AW-PID 3/integrator2 ==
  in_1 : Inport
  umax : Inport  Port=2
  umin : Inport  Port=3
  init flag : Inport  Port=4
  init val : Inport  Port=5
  Data Type Conversion : DataTypeConversion  OutDataTypeMode=int16  SaturateOnIntegerOverflow=on  RndMeth=Zero
  Data Type Conversion1 : DataTypeConversion  OutDataTypeMode=int16  SaturateOnIntegerOverflow=on  RndMeth=Zero
  Relational Operator : RelationalOperator  Operator===  InputSameDT=on
  Relational Operator1 : RelationalOperator  Operator===  InputSameDT=on
  Switch : Switch  SaturateOnIntegerOverflow=on  InputSameDT=on
  Switch1 : Switch  SaturateOnIntegerOverflow=on  InputSameDT=on
  Switch2 : Switch  SaturateOnIntegerOverflow=on  InputSameDT=on
  Unit Delay : UnitDelay  Orientation=left  SampleTime=DT
  error1 : Sum  Inputs=+++  SaturateOnIntegerOverflow=on  InputSameDT=on
  error2 : Sum  Inputs=-+  SaturateOnIntegerOverflow=on  InputSameDT=on
  error3 : Sum  Inputs=+-  SaturateOnIntegerOverflow=on  InputSameDT=on
  error4 : Sum  Inputs=+-  SaturateOnIntegerOverflow=on  InputSameDT=on
  gain : Gain  Gain=DT  SaturateOnIntegerOverflow=on
  gain1 : Gain  Orientation=left  Gain=DT*pole  SaturateOnIntegerOverflow=on
  out_1 : Outport  InitialOutput=0
  out_2 : Outport  Port=2  InitialOutput=0
  wires:
  Data Type Conversion1/1 -> error4/2
  Data Type Conversion/1 -> error4/1
  Unit Delay/1 -> gain1/1, error1/1
  error4/1 -> out_2/1
  Relational Operator/1 -> Data Type Conversion/1
  Relational Operator1/1 -> Data Type Conversion1/1
  Switch/1 -> Switch2/1, error3/1
  init val/1 -> Switch1/3
  init flag/1 -> Switch1/2
  Switch2/1 -> Relational Operator1/1, Relational Operator/1, Switch1/1
  Switch1/1 -> Unit Delay/1, out_1/1
  gain1/1 -> error1/2
  gain/1 -> error1/3
  error2/1 -> Switch/2
  error3/1 -> Switch2/2
  umin/1 -> Relational Operator1/2, error3/2, Switch2/3
  umax/1 -> Relational Operator/2, error2/2, Switch/3
  error1/1 -> error2/1, Switch/1
  in_1/1 -> gain/1

== system cblocks/AW-PID 3/variable saturation ==
  in_1 : Inport
  umax : Inport  Port=2
  umin : Inport  Port=3
  Switch : Switch  SaturateOnIntegerOverflow=on  InputSameDT=on
  Switch2 : Switch  SaturateOnIntegerOverflow=on  InputSameDT=on
  error2 : Sum  Inputs=+-  SaturateOnIntegerOverflow=on  InputSameDT=on
  error3 : Sum  Inputs=+-  SaturateOnIntegerOverflow=on  InputSameDT=on
  out_1 : Outport  InitialOutput=0
  wires:
  in_1/1 -> Switch/1, error2/2
  Switch2/1 -> out_1/1
  Switch/1 -> Switch2/1, error3/1
  umax/1 -> Switch/3, error2/1
  umin/1 -> Switch2/3, error3/2
  error3/1 -> Switch2/2
  error2/1 -> Switch/2

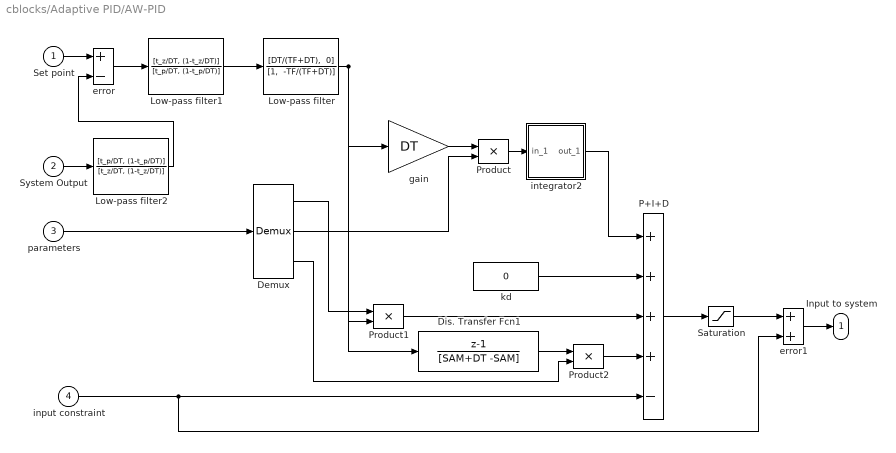
== system cblocks/Adaptive PID/AW-PID  ==
  Set point : Inport
  System Output : Inport  Port=2
  parameters : Inport  Port=3
  input constraint : Inport  Port=4
  Demux : Demux  Outputs=3
  Dis. Transfer Fcn1 : DiscreteTransferFcn  Numerator=[1 -1]  Denominator=[SAM+DT -SAM]  SampleTime=DT
  Low-pass filter : DiscreteTransferFcn  Numerator="[DT/(TF+DT),  0]"  Denominator="[1,  -TF/(TF+DT)]"  SampleTime=DT
  Low-pass filter1 : DiscreteTransferFcn  Numerator=[t_z/DT, (1-t_z/DT)]  Denominator=[t_p/DT, (1-t_p/DT)]  SampleTime=DT
  Low-pass filter2 : DiscreteTransferFcn  Numerator=[t_p/DT, (1-t_p/DT)]  Denominator=[t_z/DT, (1-t_z/DT)]  SampleTime=DT
  P+I+D : Sum  Inputs=++++-  SaturateOnIntegerOverflow=on  InputSameDT=on
  Product : Product  SaturateOnIntegerOverflow=on  InputSameDT=on
  Product1 : Product  SaturateOnIntegerOverflow=on  InputSameDT=on
  Product2 : Product  SaturateOnIntegerOverflow=on  InputSameDT=on
  Saturation : Saturate  UpperLimit=umax  LowerLimit=umin
  error : Sum  Inputs=+-  SaturateOnIntegerOverflow=on  InputSameDT=on
  error1 : Sum  SaturateOnIntegerOverflow=on  InputSameDT=on
  gain : Gain  Gain=DT  SaturateOnIntegerOverflow=on
  integrator2 : Subsystem  mask(Anti windup intgrator){@1=umax, @2=umin, @3=DT}
      mask prompts: @1 "umax"; @2 "umin"; @3 "sampling time"
      mask help: Integral with anti-windup
      mask init:
      | umax=@1 ; umin =@2 ;DT=@3;
      mask Display: disp('DT-I-AW')
  kd : Constant  Value=0  OutDataType=sfix(16)  ConRadixGroup=Use specified scaling  OutScaling=2^0  SampleTime=inf  FramePeriod=inf
  Input to system : Outport  InitialOutput=0
  wires:
  Set point/1 -> error/1
  parameters/1 -> Demux/1
  input constraint/1 -> P+I+D/5, error1/2
  error/1 -> Low-pass filter1/1
  integrator2/1(out_1) -> P+I+D/1
  Low-pass filter/1 -> Product1/2, gain/1, Dis. Transfer Fcn1/1
  Product1/1 -> P+I+D/3
  P+I+D/1 -> Saturation/1
  Product/1 -> integrator2/1(in_1)
  gain/1 -> Product/1
  Demux/1 -> Product1/1
  Demux/2 -> Product/2
  Saturation/1 -> error1/1
  error1/1 -> Input to system/1
  Product2/1 -> P+I+D/4
  Dis. Transfer Fcn1/1 -> Product2/1
  Demux/3 -> Product2/2
  kd/1 -> P+I+D/2
  Low-pass filter1/1 -> Low-pass filter/1
  System Output/1 -> Low-pass filter2/1
  Low-pass filter2/1 -> error/2

== system cblocks/Adaptive PID/Inner Product ==
  in_1 : Inport
  in_2 : Inport  Port=2
  Product : Product  SaturateOnIntegerOverflow=on  InputSameDT=on
  Sum : Sum  Inputs=+  SaturateOnIntegerOverflow=on  InputSameDT=on
  out_1 : Outport  InitialOutput=0
  wires:
  Sum/1 -> out_1/1
  Product/1 -> Sum/1
  in_1/1 -> Product/1
  in_2/1 -> Product/2

== system cblocks/Adaptive PID/Inner Product1 ==
  in_1 : Inport
  in_2 : Inport  Port=2
  Product : Product  SaturateOnIntegerOverflow=on  InputSameDT=on
  Sum : Sum  Inputs=+  SaturateOnIntegerOverflow=on  InputSameDT=on
  out_1 : Outport  InitialOutput=0
  wires:
  Sum/1 -> out_1/1
  Product/1 -> Sum/1
  in_1/1 -> Product/1
  in_2/1 -> Product/2

== system cblocks/Adaptive PID/Inner Product2 ==
  in_1 : Inport
  in_2 : Inport  Port=2
  Product : Product  SaturateOnIntegerOverflow=on  InputSameDT=on
  Sum : Sum  Inputs=+  SaturateOnIntegerOverflow=on  InputSameDT=on
  out_1 : Outport  InitialOutput=0
  wires:
  Sum/1 -> out_1/1
  Product/1 -> Sum/1
  in_1/1 -> Product/1
  in_2/1 -> Product/2

== system cblocks/MIMO controller st-sp+AW/feedback filter ==
  in_1 : Inport
  A : StateSpace  A=[]  B=[]  C=[]  D=K  mask(Matrix Gain){@1=Afo}
      mask prompts: @1 "Gain matrix:"
      mask help: Matrix Gain.
      mask init:
      | K = @1;
      mask Help: Multiplies input vector by entered matrix to produce output vector (y=Au).
      mask Display: disp('K')
  B : StateSpace  A=[]  B=[]  C=[]  D=K  mask(Matrix Gain){@1=Bfo}
      mask prompts: @1 "Gain matrix:"
      mask help: Matrix Gain.
      mask init:
      | K = @1;
      mask Help: Multiplies input vector by entered matrix to produce output vector (y=Au).
      mask Display: disp('K')
  C : StateSpace  A=[]  B=[]  C=[]  D=K  mask(Matrix Gain){@1=Cfo}
      mask prompts: @1 "Gain matrix:"
      mask help: Matrix Gain.
      mask init:
      | K = @1;
      mask Help: Multiplies input vector by entered matrix to produce output vector (y=Au).
      mask Display: disp('K')
  D : StateSpace  A=[]  B=[]  C=[]  D=K  mask(Matrix Gain){@1=Dfo}
      mask prompts: @1 "Gain matrix:"
      mask help: Matrix Gain.
      mask init:
      | K = @1;
      mask Help: Multiplies input vector by entered matrix to produce output vector (y=Au).
      mask Display: disp('K')
  Sum1 : Sum  SaturateOnIntegerOverflow=on  InputSameDT=on
  Sum2 : Sum  SaturateOnIntegerOverflow=on  InputSameDT=on
  Unit Delay : UnitDelay  SampleTime=TSAMPLE
  out_1 : Outport  InitialOutput=0
  wires:
  Unit Delay/1 -> C/1, A/1
  C/1 -> Sum1/2
  B/1 -> Sum2/2
  A/1 -> Sum2/1
  Sum2/1 -> Unit Delay/1
  Sum1/1 -> out_1/1
  D/1 -> Sum1/1
  in_1/1 -> D/1, B/1

== system cblocks/MIMO controller st-sp+AW/satur ==
  in_1 : Inport
  Saturation1 : Saturate  UpperLimit=Upmax  LowerLimit=Upmin
  Sum2 : Sum  Inputs=-+  SaturateOnIntegerOverflow=on  InputSameDT=on
  out_1 : Outport  InitialOutput=0
  out_2 : Outport  Port=2  InitialOutput=0
  wires:
  Saturation1/1 -> out_1/1, Sum2/1
  Sum2/1 -> out_2/1
  in_1/1 -> Sum2/2, Saturation1/1

== system cblocks/MIMO controller st-sp+AW1/feedback filter ==
  in_1 : Inport
  A : StateSpace  A=[]  B=[]  C=[]  D=K  mask(Matrix Gain){@1=Afo}
      mask prompts: @1 "Gain matrix:"
      mask help: Matrix Gain.
      mask init:
      | K = @1;
      mask Help: Multiplies input vector by entered matrix to produce output vector (y=Au).
      mask Display: disp('K')
  B : StateSpace  A=[]  B=[]  C=[]  D=K  mask(Matrix Gain){@1=Bfo}
      mask prompts: @1 "Gain matrix:"
      mask help: Matrix Gain.
      mask init:
      | K = @1;
      mask Help: Multiplies input vector by entered matrix to produce output vector (y=Au).
      mask Display: disp('K')
  C : StateSpace  A=[]  B=[]  C=[]  D=K  mask(Matrix Gain){@1=Cfo}
      mask prompts: @1 "Gain matrix:"
      mask help: Matrix Gain.
      mask init:
      | K = @1;
      mask Help: Multiplies input vector by entered matrix to produce output vector (y=Au).
      mask Display: disp('K')
  D : StateSpace  A=[]  B=[]  C=[]  D=K  mask(Matrix Gain){@1=Dfo}
      mask prompts: @1 "Gain matrix:"
      mask help: Matrix Gain.
      mask init:
      | K = @1;
      mask Help: Multiplies input vector by entered matrix to produce output vector (y=Au).
      mask Display: disp('K')
  Sum1 : Sum  SaturateOnIntegerOverflow=on  InputSameDT=on
  Sum2 : Sum  SaturateOnIntegerOverflow=on  InputSameDT=on
  Unit Delay : UnitDelay  SampleTime=TSAMPLE
  out_1 : Outport  InitialOutput=0
  wires:
  Unit Delay/1 -> C/1, A/1
  C/1 -> Sum1/2
  B/1 -> Sum2/2
  A/1 -> Sum2/1
  Sum2/1 -> Unit Delay/1
  Sum1/1 -> out_1/1
  D/1 -> Sum1/1
  in_1/1 -> D/1, B/1

== system cblocks/MIMO controller st-sp+AW1/satur ==
  in_1 : Inport
  Saturation1 : Saturate  UpperLimit=Upmax  LowerLimit=Upmin
  Sum2 : Sum  Inputs=-+  SaturateOnIntegerOverflow=on  InputSameDT=on
  out_1 : Outport  InitialOutput=0
  out_2 : Outport  Port=2  InitialOutput=0
  wires:
  Saturation1/1 -> out_1/1, Sum2/1
  Sum2/1 -> out_2/1
  in_1/1 -> Sum2/2, Saturation1/1

== system cblocks/MIMO controller st-sp+AW2/feedback filter ==
  in_1 : Inport
  A : StateSpace  A=[]  B=[]  C=[]  D=K  mask(Matrix Gain){@1=Afo}
      mask prompts: @1 "Gain matrix:"
      mask help: Matrix Gain.
      mask init:
      | K = @1;
      mask Help: Multiplies input vector by entered matrix to produce output vector (y=Au).
      mask Display: disp('K')
  B : StateSpace  A=[]  B=[]  C=[]  D=K  mask(Matrix Gain){@1=Bfo}
      mask prompts: @1 "Gain matrix:"
      mask help: Matrix Gain.
      mask init:
      | K = @1;
      mask Help: Multiplies input vector by entered matrix to produce output vector (y=Au).
      mask Display: disp('K')
  C : StateSpace  A=[]  B=[]  C=[]  D=K  mask(Matrix Gain){@1=Cfo}
      mask prompts: @1 "Gain matrix:"
      mask help: Matrix Gain.
      mask init:
      | K = @1;
      mask Help: Multiplies input vector by entered matrix to produce output vector (y=Au).
      mask Display: disp('K')
  D : StateSpace  A=[]  B=[]  C=[]  D=K  mask(Matrix Gain){@1=Dfo}
      mask prompts: @1 "Gain matrix:"
      mask help: Matrix Gain.
      mask init:
      | K = @1;
      mask Help: Multiplies input vector by entered matrix to produce output vector (y=Au).
      mask Display: disp('K')
  Sum1 : Sum  SaturateOnIntegerOverflow=on  InputSameDT=on
  Sum2 : Sum  SaturateOnIntegerOverflow=on  InputSameDT=on
  Unit Delay : UnitDelay  SampleTime=TSAMPLE
  out_1 : Outport  InitialOutput=0
  wires:
  Unit Delay/1 -> C/1, A/1
  C/1 -> Sum1/2
  B/1 -> Sum2/2
  A/1 -> Sum2/1
  Sum2/1 -> Unit Delay/1
  Sum1/1 -> out_1/1
  D/1 -> Sum1/1
  in_1/1 -> D/1, B/1

== system cblocks/MIMO controller st-sp+AW2/satur ==
  u_desired : Inport
  ys : Inport  Port=2
  Saturation1 : Saturate  UpperLimit=Upmax  LowerLimit=Upmin
  Sum1 : Sum  Inputs=+-  SaturateOnIntegerOverflow=on  InputSameDT=on
  Sum2 : Sum  Inputs=+-  SaturateOnIntegerOverflow=on  InputSameDT=on
  Sum3 : Sum  Inputs=+-  SaturateOnIntegerOverflow=on  InputSameDT=on
  Unit Delay1 : UnitDelay  SampleTime=TSAMPLE
  plant model : Subsystem
  power : Outport
  ysadjust : Outport  Port=2
  wires:
  Saturation1/1 -> power/1, Sum2/1
  u_desired/1 -> Sum2/2, Sum3/1
  Sum2/1 -> plant model/1(in_1)
  ys/1 -> Sum1/1
  plant model/1(spike) -> Sum1/2
  plant model/2(out_2) -> Sum3/2
  Sum3/1 -> Saturation1/1
  Sum1/1 -> Unit Delay1/1
  Unit Delay1/1 -> ysadjust/1

== system cblocks/standard PID/integrator1 ==
  in_1 : Inport
  delay : DiscreteTransferFcn  Orientation=left  Denominator=[1 0]  SampleTime=DT
  error1 : Sum  SaturateOnIntegerOverflow=on  InputSameDT=on
  out_1 : Outport  InitialOutput=0
  wires:
  in_1/1 -> error1/2
  error1/1 -> out_1/1, delay/1
  delay/1 -> error1/1

== system cblocks/Adaptive PID/AW-PID /integrator2 ==
  in_1 : Inport
  Constant : Constant  Value=umax  OutDataType=sfix(16)  ConRadixGroup=Use specified scaling  OutScaling=2^0  SampleTime=inf  FramePeriod=inf
  Constant3 : Constant  Value=umin  OutDataType=sfix(16)  ConRadixGroup=Use specified scaling  OutScaling=2^0  SampleTime=inf  FramePeriod=inf
  Switch : Switch  SaturateOnIntegerOverflow=on  InputSameDT=on
  Switch2 : Switch  SaturateOnIntegerOverflow=on  InputSameDT=on
  delay : DiscreteTransferFcn  Orientation=left  Denominator=[1 0]  SampleTime=DT
  error1 : Sum  SaturateOnIntegerOverflow=on  InputSameDT=on
  error2 : Sum  Inputs=+-  SaturateOnIntegerOverflow=on  InputSameDT=on
  error3 : Sum  Inputs=+-  SaturateOnIntegerOverflow=on  InputSameDT=on
  out_1 : Outport  InitialOutput=0
  wires:
  delay/1 -> error1/1
  error2/1 -> Switch/2
  error3/1 -> Switch2/2
  Constant3/1 -> error3/2, Switch2/3
  Constant/1 -> error2/1, Switch/3
  error1/1 -> error2/2, Switch/1
  Switch/1 -> error3/1, Switch2/1
  Switch2/1 -> delay/1, out_1/1
  in_1/1 -> error1/2

== system cblocks/MIMO controller st-sp+AW2/satur/plant model ==
  in_1 : Inport
  A : StateSpace  A=[]  B=[]  C=[]  D=K  mask(Matrix Gain){@1=A_td}
      mask prompts: @1 "Gain matrix:"
      mask help: Matrix Gain.
      mask init:
      | K = @1;
      mask Help: Multiplies input vector by entered matrix to produce output vector (y=Au).
      mask Display: disp('K')
  B : StateSpace  A=[]  B=[]  C=[]  D=K  mask(Matrix Gain){@1=B_td}
      mask prompts: @1 "Gain matrix:"
      mask help: Matrix Gain.
      mask init:
      | K = @1;
      mask Help: Multiplies input vector by entered matrix to produce output vector (y=Au).
      mask Display: disp('K')
  C1 : StateSpace  A=[]  B=[]  C=[]  D=K  mask(Matrix Gain){@1=K_td}
      mask prompts: @1 "Gain matrix:"
      mask help: Matrix Gain.
      mask init:
      | K = @1;
      mask Help: Multiplies input vector by entered matrix to produce output vector (y=Au).
      mask Display: disp('K')
  Cs : StateSpace  A=[]  B=[]  C=[]  D=K  mask(Matrix Gain){@1=C_td}
      mask prompts: @1 "Gain matrix:"
      mask help: Matrix Gain.
      mask init:
      | K = @1;
      mask Help: Multiplies input vector by entered matrix to produce output vector (y=Au).
      mask Display: disp('K')
  Ds : StateSpace  A=[]  B=[]  C=[]  D=K  mask(Matrix Gain){@1=D_td}
      mask prompts: @1 "Gain matrix:"
      mask help: Matrix Gain.
      mask init:
      | K = @1;
      mask Help: Multiplies input vector by entered matrix to produce output vector (y=Au).
      mask Display: disp('K')
  Sum1 : Sum  SaturateOnIntegerOverflow=on  InputSameDT=on
  Sum2 : Sum  SaturateOnIntegerOverflow=on  InputSameDT=on
  Unit Delay : UnitDelay  SampleTime=TSAMPLE
  spike : Outport
  out_2 : Outport  Port=2
  wires:
  in_1/1 -> Ds/1, B/1
  Unit Delay/1 -> A/1, C1/1, Cs/1
  Ds/1 -> Sum1/1
  Sum2/1 -> Unit Delay/1
  A/1 -> Sum2/1
  B/1 -> Sum2/2
  Cs/1 -> Sum1/2
  Sum1/1 -> spike/1
  C1/1 -> out_2/1
